simulink model "PID_REFERENCE_MODEL"  (R2020b)
settings: Solver=VariableStepAuto  StartTime=0.0  StopTime=10  RelTol=1e-3
model mask{kd=170.553062, ki=289087.103, kp=14418.122}
PreLoadFcn:
  | vars
model workspace (MAT data in the model file):
  kd = 170.553062
  ki = 289087.103
  kp = 14418.122
settings Model: DataDictionary=problem_DD.sldd  ParameterArgumentNames=kd,ki,kp  Creator=hp  LastModifiedBy=hp
settings DataIOCC: SaveOutput=off  SaveTime=off

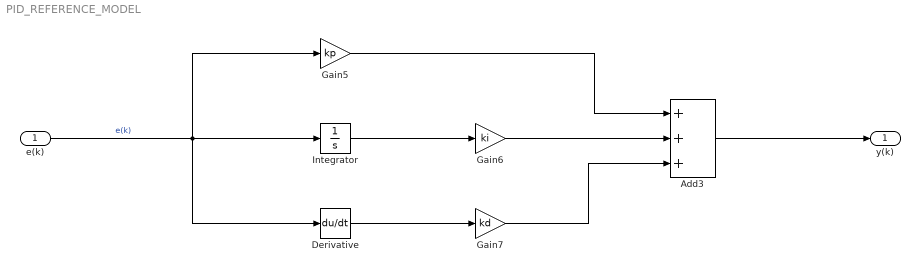
== system PID_REFERENCE_MODEL ==
  e(k) : Inport  OutDataTypeStr=double  PortDimensions=1  SampleTime=0
  Add3 : Sum  Inputs=+++
  Derivative : Derivative
  Gain5 : Gain  Gain=kp
  Gain6 : Gain  Gain=ki
  Gain7 : Gain  Gain=kd
  Integrator : Integrator
  y(k) : Outport  OutDataTypeStr=double  PortDimensions=1  SampleTime=0
  wires:
  Derivative/1 -> Gain7/1
  e(k)/1 -> Gain5/1, Integrator/1, Derivative/1  "e(k)"
  Integrator/1 -> Gain6/1
  Gain7/1 -> Add3/3
  Gain6/1 -> Add3/2
  Gain5/1 -> Add3/1
  Add3/1 -> y(k)/1
